simulink model "buck_protection_state_machine_logic"  (R2024b)
settings: Solver=FixedStepDiscrete  StartTime=0.0  StopTime=0.018  FixedStep=5e-5  RelTol=1e-3
settings Model: Creator=ww  LastModifiedBy=ww

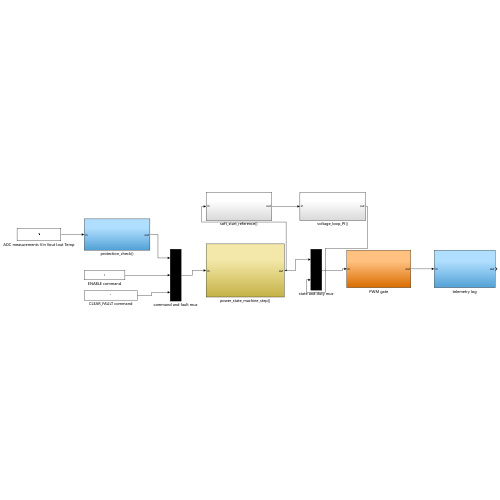
[thumbnail: Simulink's stored preview of the top-level diagram]
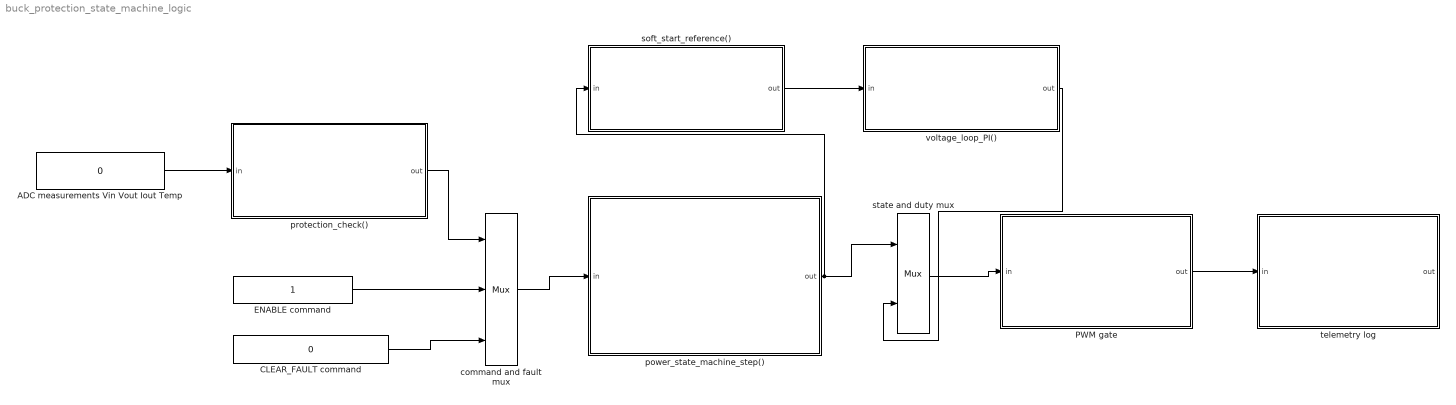
== system buck_protection_state_machine_logic ==
  ADC measurements Vin Vout Iout Temp : Constant  Value=0
  CLEAR_FAULT command : Constant  Value=0
  ENABLE command : Constant
  PWM gate : Subsystem
  command and fault mux : Mux  Inputs=3
  power_state_machine_step() : Subsystem
  protection_check() : Subsystem
  soft_start_reference() : Subsystem
  state and duty mux : Mux  Inputs=2
  telemetry log : Subsystem
  voltage_loop_PI() : Subsystem
  wires:
  ADC measurements Vin Vout Iout Temp/1 -> protection_check()/1(in)
  protection_check()/1(out) -> command and fault mux/1
  ENABLE command/1 -> command and fault mux/2
  CLEAR_FAULT command/1 -> command and fault mux/3
  command and fault mux/1 -> power_state_machine_step()/1(in)
  power_state_machine_step()/1(out) -> soft_start_reference()/1(in), state and duty mux/1
  soft_start_reference()/1(out) -> voltage_loop_PI()/1(in)
  voltage_loop_PI()/1(out) -> state and duty mux/2
  state and duty mux/1 -> PWM gate/1(in)
  PWM gate/1(out) -> telemetry log/1(in)

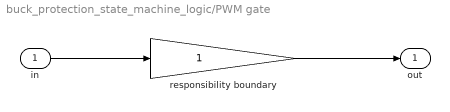
== system buck_protection_state_machine_logic/PWM gate ==
  in : Inport
  responsibility boundary : Gain  Description=|
      | RUN/SOFT_START: pass duty
      | IDLE/FAULT/RECOVERY: duty=0
      | Single PWM shutdown exit
  out : Outport
  wires:
  in/1 -> responsibility boundary/1
  responsibility boundary/1 -> out/1

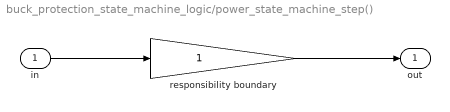
== system buck_protection_state_machine_logic/power_state_machine_step() ==
  in : Inport
  responsibility boundary : Gain  Description=|
      | INIT -> IDLE
      | IDLE -> SOFT_START
      | SOFT_START -> RUN
      | fault -> FAULT_LATCH
      | clear -> RECOVERY -> IDLE
  out : Outport
  wires:
  in/1 -> responsibility boundary/1
  responsibility boundary/1 -> out/1

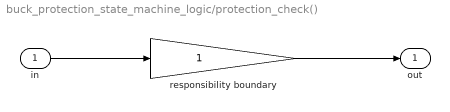
== system buck_protection_state_machine_logic/protection_check() ==
  in : Inport
  responsibility boundary : Gain  Description=|
      | OCP: Iout > threshold
      | OVP: Vout > threshold
      | UVLO: Vin < threshold
      | OTP: Temp > threshold
      | Output: one fault code
  out : Outport
  wires:
  in/1 -> responsibility boundary/1
  responsibility boundary/1 -> out/1

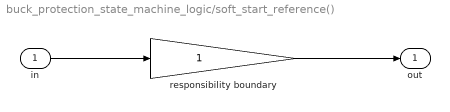
== system buck_protection_state_machine_logic/soft_start_reference() ==
  in : Inport
  responsibility boundary : Gain  Description=|
      | Runs only in SOFT_START
      | Generates Vref_cmd ramp
      | Does not decide faults
  out : Outport
  wires:
  in/1 -> responsibility boundary/1
  responsibility boundary/1 -> out/1

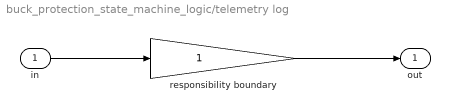
== system buck_protection_state_machine_logic/telemetry log ==
  in : Inport
  responsibility boundary : Gain  Description=|
      | state
      | detected fault
      | latched fault
      | PWM enable
      | duty cmd
  out : Outport
  wires:
  in/1 -> responsibility boundary/1
  responsibility boundary/1 -> out/1

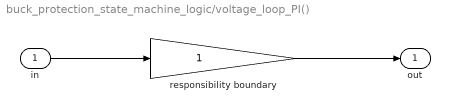
== system buck_protection_state_machine_logic/voltage_loop_PI() ==
  in : Inport
  responsibility boundary : Gain  Description=|
      | Input: Vref_cmd and Vout
      | Output: duty candidate
      | No fault threshold checks
  out : Outport
  wires:
  in/1 -> responsibility boundary/1
  responsibility boundary/1 -> out/1
